simulink model "sm_DDPG_Training_Circuit_h4"  (R2022b)
settings: Solver=VariableStepAuto  StartTime=0.0  StopTime=2000  RelTol=1e-3
values from neighbouring files (symbols this model uses):
  areaFinEvap = 0.05    [pramInit.m]
  areaRoofRoom1 = roofArea/4    [pramInit.m]
  areaRoofRoom2 = roofArea/4    [pramInit.m]
  areaRoofRoom3 = roofArea/4    [pramInit.m]
  areaRoofRoom4 = roofArea/4    [pramInit.m]
  areaWallRoom1 = (lenHouse*3/5 *htHouse+widHouse*2/3*htHouse) - areaWindowRoom1    (= 95.6666666667)    [pramInit.m]
  areaWallRoom2 = (lenHouse*3/5*htHouse+widHouse/3*htHouse) - areaWindowRoom2    (= 83.3333333333)    [pramInit.m]
  areaWallRoom3 = (lenHouse*2/5*htHouse+widHouse*2/3*htHouse) - areaWindowRoom3    (= 72.6666666667)    [pramInit.m]
  areaWallRoom4 = (lenHouse*2/5*htHouse+widHouse/3*htHouse) - areaWindowRoom4    (= 59.3333333333)    [pramInit.m]
  areaWindowRoom1 = 3 * 1 *1    (= 3)    [pramInit.m]
  areaWindowRoom2 = 2 * 1 *1    (= 2)    [pramInit.m]
  areaWindowRoom3 = 2* 1 *1    (= 2)    [pramInit.m]
  areaWindowRoom4 = 2 * 1 *1    (= 2)    [pramInit.m]
  diaCond = 0.014    [pramInit.m]
  diaEvap = 0.126    [pramInit.m]
  diaGroundLoop = 0.032    [pramInit.m]
  diaOuterCond = 0.0158    [pramInit.m]
  diaOuterEvap = 0.1344    [pramInit.m]
  diaRadiatorPipe = 0.0125    [pramInit.m]
  htCondDuct = 0.3    [pramInit.m]
  htEvapDuct = 2.5    [pramInit.m]
  kTube = 400    [pramInit.m]
  leakRoofPercent = 0.1    [pramInit.m]
  leakWallPercent = 0.15    [pramInit.m]
  leakWinPercent = 0.2    [pramInit.m]
  numFinsEvap = 90    [pramInit.m]
  numTubeRowsCond = 20    [pramInit.m]
  numTubeRowsEvap = 400    [pramInit.m]
  numTubesPerRowCond = 10    [pramInit.m]
  numTubesPerRowEvap = 20    [pramInit.m]
  qGroundLoopPump = 18    [pramInit.m]
  roofDensity = 32    [pramInit.m]
  thkRoof = 0.2    [pramInit.m]
  thkWall = 0.2    [pramInit.m]
  thkWindow = 0.01    [pramInit.m]
  tInitHW = 50    [pramInit.m]
  tRoom = 23    [pramInit.m]
  Ts = hyper_agent_sample_time    [code_DDPG_Training.m]    (also in code_Experimental_Setup.m = 1)
  wallDensity = 1920    [pramInit.m]
  wCondDuct = 1.6    [pramInit.m]
  wEvapDuct = 0.96    [pramInit.m]
  windowDensity = 2700    [pramInit.m]
undefined symbols (not defined in the file or in its folder): DiscIntNeverNeededParam
libraries: fl_lib x144, nesl_utility x27, SimscapeFluids_lib x15, simulink x3, rllib x1
(part 1 of 4)
settings Model: Creator=rajeshs  LastModifiedBy=xmyci
settings SolverCC: AlgebraicLoopSolver=LineSearch
settings DebuggingCC: UnconnectedInputMsg=warning  UnconnectedOutputMsg=warning  UnconnectedLineMsg=warning  SFMachineParentedDataDiag=warning
settings ModelReferenceCC: EnableRefExpFcnMdlSchedulingChecks=on
settings SFSimCC: CustomCodeUndefinedFunction=UseInterfaceOnly
settings RTWCC: DLArmComputeVersion=19.05

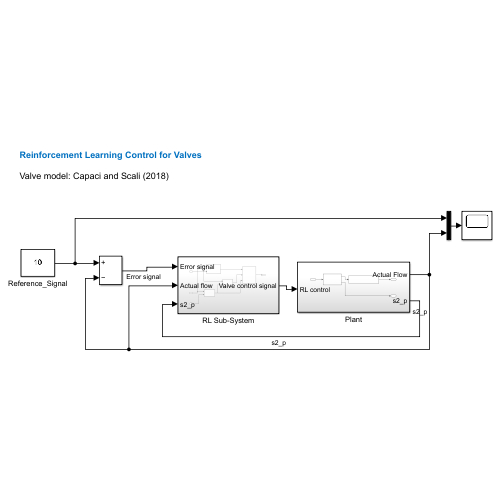
[thumbnail: Simulink's stored preview of the top-level diagram]
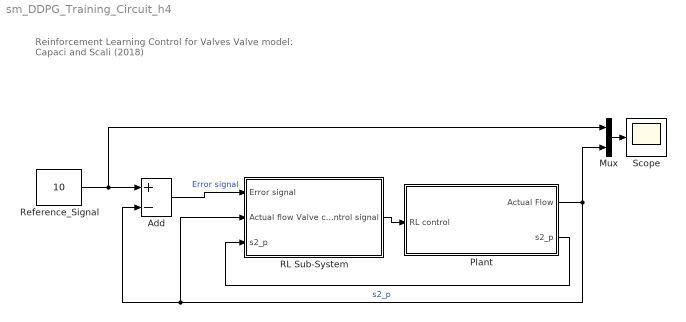
== system sm_DDPG_Training_Circuit_h4 ==
  note: Reinforcement Learning Control for Valves
      |
      | Valve model: Capaci and Scali (2018)
  Add : Sum  Inputs=+-
  Mux : Mux  Inputs=2
  Plant : Subsystem
  RL Sub-System : Subsystem
  Reference_Signal : Constant  Value=10
  Scope : Scope
  wires:
  Mux/1 -> Scope/1
  Add/1 -> RL Sub-System/1(Error signal)  "Error signal"
  Plant/1(Actual Flow) -> Add/2, RL Sub-System/2(Actual flow), Mux/2  "s2_p"
  Reference_Signal/1 -> Mux/1, Add/1
  RL Sub-System/1(Valve control signal) -> Plant/1(RL control)
  Plant/2(s2_p) -> RL Sub-System/3(s2_p)

== system sm_DDPG_Training_Circuit_h4/Plant ==
  RL control : Inport
  Non-linear Valve model : Subsystem
  Process : Subsystem
  Actual Flow : Outport  VectorParamsAs1DForOutWhenUnconnected=off
  s2_p : Outport  Port=2  VectorParamsAs1DForOutWhenUnconnected=off
  wires:
  Non-linear Valve model/1(ValveOutput) -> Process/1(Valve control)
  Process/1(Controlled_Flow) -> Actual Flow/1  "Actual Flow"
  RL control/1 -> Non-linear Valve model/1(ValveInput)
  Non-linear Valve model/2(S2_p) -> s2_p/1  "s2_p"

== system sm_DDPG_Training_Circuit_h4/RL Sub-System ==
  Error signal : Inport
  Actual flow : Inport  Port=2
  s2_p : Inport  Port=3
  Compute Rewards : Subsystem
  Observation vector : Subsystem
  RL Agent : rllib/RL Agent  Agent=agent  ExternalActionAsInput=off  ProvideLastAction=off  ProvideCumRwd=off  TreatAsDirectFeedthrough=on  UseStrictObservationDataTypes=off
  Stop-simulation : Subsystem
  Valve control signal : Outport  VectorParamsAs1DForOutWhenUnconnected=off
  wires:
  Stop-simulation/1(STOP) -> RL Agent/3, Compute Rewards/2(exceeds flow)
  Error signal/1 -> Compute Rewards/1(error), Observation vector/2(Error signal)
  Compute Rewards/1(reward) -> RL Agent/2
  Observation vector/1(Observation vector) -> RL Agent/1
  RL Agent/1 -> Valve control signal/1
  Actual flow/1 -> Observation vector/1(Actual flow), Stop-simulation/1(Actual flow)
  s2_p/1 -> Stop-simulation/2(s2_p)

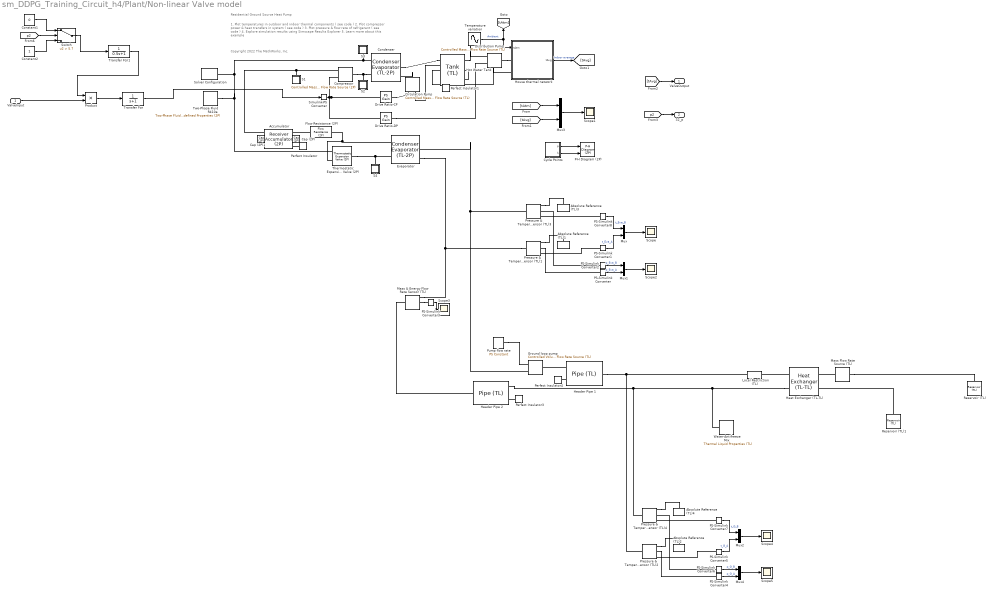
== system sm_DDPG_Training_Circuit_h4/Plant/Non-linear Valve model ==
  note: Copyright 2022 The MathWorks, Inc.
  note: Residential Ground Source Heat Pump
  note: 1. Plot temperatures in outdoor and indoor thermal components ( see code )
      | 2. Plot compressor power & heat transfers in system ( see code )
      | 3. Plot pressure & flow rate of refrigerant ( see code )
      | 4. Explore simulation results using Simscape Results Explorer
      | 5. Learn more about this example
  ValveInput : Inport
  Absolute Reference (TL){1..4} (4 alike) : fl_lib/Thermal Liquid/Elements/Absolute Reference (TL)
  Accumulator : SimscapeFluids_lib/Two-Phase Fluid/Tanks & Accumulators/Receiver Accumulator (2P)  volume=0.02 m^3  tank_area=0.5 m^2  area_AV=pi * diaEvap^2 / 4 m^2  area_BV=pi * diaEvap^2 / 4 m^2  area_AL=pi * diaEvap^2 / 4 m^2  area_BL=pi * diaEvap^2 / 4 m^2  V_frac_error=simscape.enum.assert.action.none  V_frac_min=0.05  V_frac_max=0.95  V_frac_smooth=0.001  p_crit_error=simscape.enum.assert.action.error  hc_vap=10 W/(m^2*K)  hc_liq=20 W/(m^2*K)  receiver_accumulator_energy_spec=fluids.two_phase_fluid.enum.receiver_accumulator_energy_spec.enthalpy  p_init=0.3 MPa  T_init=293.15 K  M_frac_init=0.5  V_frac_init=0.1 %L_init  h_init=436 kJ/kg  u_init=1500 kJ/kg  tau_vap_cond=1 s
      settings: InternalSimscapePortConfiguration="{\"Bottom\":[],\"Left\":[{\"id\":\"AV\",\"label\":\"AV\",\"type\":\"foundation.two_phase_fluid.two_phase_fluid\"},{\"id\":\"AL\",\"label\":\"AL\",\"type\":\"foundation.two_phase_fluid.two_phase_fluid\"},{\"id\":\"H\",\"label\":\"H\",\"type\":\"foundation.thermal.thermal\"}],\"Right\":[{\"id\":\"BV\",\"label\":\"BV\",\"type\":\"foundation.two_phase_fluid.two_phase_fluid\"},{\"id\":\"BL\",\"label\":\"BL\",\"type\":\"foundation.two_phase_fluid.two_phase_fluid\"},{\"id\":\"L\",\"label\":\"L\",\"type\":\"output\"}],\"Top\":[]}"
  Cap (2P) : fl_lib/Two-Phase Fluid/Elements/Cap (2P)  p_specify=off  p_priority=None  p=0.101325 MPa  p_nominal_specify=off  p_nominal_unit=MPa  p_nominal_value=1  u_specify=off  u_priority=None  u=1500 kJ/kg  u_nominal_specify=off  u_nominal_unit=kJ/kg  u_nominal_value=1
      settings: InternalSimscapePortConfiguration="{\"Bottom\":[],\"Left\":[{\"id\":\"A\",\"label\":\"\",\"type\":\"foundation.two_phase_fluid.two_phase_fluid\"}],\"Right\":[],\"Top\":[]}"
  Cap (2P)1 : fl_lib/Two-Phase Fluid/Elements/Cap (2P)  p_specify=off  p_priority=None  p=0.101325 MPa  p_nominal_specify=off  p_nominal_unit=MPa  p_nominal_value=1  u_specify=off  u_priority=None  u=1500 kJ/kg  u_nominal_specify=off  u_nominal_unit=kJ/kg  u_nominal_value=1
      settings: InternalSimscapePortConfiguration="{\"Bottom\":[],\"Left\":[{\"id\":\"A\",\"label\":\"\",\"type\":\"foundation.two_phase_fluid.two_phase_fluid\"}],\"Right\":[],\"Top\":[]}"
  Circulation Pump : fl_lib/Thermal Liquid/Sources/Controlled Mass Flow Rate Source (TL)  area=0.01 m^2
      settings: InternalSimscapePortConfiguration="{\"Bottom\":[],\"Left\":[{\"id\":\"A\",\"label\":\"A\",\"type\":\"foundation.thermal_liquid.thermal_liquid\"},{\"id\":\"M\",\"label\":\"M\",\"type\":\"input\"}],\"Right\":[{\"id\":\"B\",\"label\":\"B\",\"type\":\"foundation.thermal_liquid.thermal_liquid\"}],\"Top\":[]}"
  Compressor : fl_lib/Two-Phase Fluid/Sources/Controlled Mass Flow Rate Source (2P)  power_spec=foundation.enum.power_spec.isentropic  area_A=pi * diaCond^2 /4 m^2  area_B=pi * diaCond^2 /4 m^2
      settings: InternalSimscapePortConfiguration="{\"Bottom\":[],\"Left\":[{\"id\":\"A\",\"label\":\"A\",\"type\":\"foundation.two_phase_fluid.two_phase_fluid\"},{\"id\":\"M\",\"label\":\"M\",\"type\":\"input\"}],\"Right\":[{\"id\":\"B\",\"label\":\"B\",\"type\":\"foundation.two_phase_fluid.two_phase_fluid\"}],\"Top\":[]}"
  Condenser : SimscapeFluids_lib/Fluid Network Interfaces/Heat Exchangers/Condenser Evaporator (TL-2P)  flow_arrangement=fluids.interfaces.heat_exchangers.enum.FlowArrangementTL2P.Counter  cross_flow_arrangement=fluids.interfaces.heat_exchangers.enum.CrossFlowArrangementTL2P.UnmixedUnmixed  R_wall=log(diaOuterCond/diaCond) / (2*pi*kTube*wCondDuct*numTubeRowsCond*numTubesPerRowCond) K/kW  area_A1=wCondDuct * htCondDuct m^2  area_B1=wCondDuct * htCondDuct m^2  area_A2=pi * diaCond^2 /4 m^2  area_B2=pi * diaCond^2 /4 m^2  flow_geometry_TL=fluids.interfaces.heat_exchangers.enum.FlowGeometryTL.AcrossTubeBank  tube_num_TL=25  tube_length_TL=1 m  tube_cross_section_TL=fluids.interfaces.heat_exchangers.enum.TubeCrossSection.Circular  tube_diameter_TL=0.05 m  tube_width_TL=0.05 m  tube_height_TL=0.05 m  tube_inner_diameter_TL=0.05 m  tube_outer_diameter_TL=0.1 m  tube_flow_area_TL=0.002 m^2  tube_wetted_perimeter_TL=0.15 m  tube_heat_perimeter_TL=0.15 m  tube_pressure_loss_spec_TL=fluids.interfaces.heat_exchangers.enum.TubePressureLossSpec.Haaland  tube_loss_coeff_TL=10  tube_length_add_TL=0.1 m  tube_roughness_pressure_TL=15e-6 m  tube_Re_lam_pressure_TL=2000  tube_Re_tur_pressure_TL=4000  tube_shape_factor_generic_TL=64  tube_heat_coeff_spec_TL=fluids.interfaces.heat_exchangers.enum.TubeHeatCoeffSpec.Gneilinski  tube_colburn_coeff_TL=[.023, .8, .33]  tube_roughness_heat_TL=15e-6 m  tube_Re_lam_heat_TL=2000  tube_Re_tur_heat_TL=4000  tube_Nu_lam_generic_TL=3.66  bank_arrangement_TL=fluids.interfaces.heat_exchangers.enum.BankArrangement.Inline  bank_num_rows_TL=numTubeRowsCond  bank_tubes_per_row_TL=numTubesPerRowCond  bank_width_TL=wCondDuct m  bank_tube_diameter_TL=diaCond m  bank_longitudinal_pitch_TL=longPitchCond m  bank_transverse_pitch_TL=transPitchCond m  bank_pressure_loss_spec_TL=fluids.interfaces.heat_exchangers.enum.BankPressureLossSpec.Martin  bank_euler_TL=10  bank_heat_coeff_spec_TL=fluids.interfaces.heat_exchangers.enum.BankHeatCoeffSpec.Martin  bank_colburn_coeff_TL=[.27, .63, .36]  generic_flow_area_TL=0.01 m^2  generic_heat_area_TL=2 m^2  generic_volume_TL=0.05 m^3  generic_loss_coeff_TL=10  generic_colburn_coeff_TL=[.023, .8, .33]  fouling_factor_TL=0.1 K*m^2/kW  fin_area_TL=0.02 m^2  fin_efficiency_TL=0.5  p_init_TL=pInitHW MPa  T_init_TL=tInitHW degC  tube_num_2P=1  tube_length_2P=wCondDuct * numTubeRowsCond * numTubesPerRowCond m  tube_cross_section_2P=fluids.interfaces.heat_exchangers.enum.TubeCrossSection.Circular  tube_diameter_2P=diaCond m  tube_width_2P=0.05 m  tube_height_2P=0.05 m  tube_inner_diameter_2P=0.05 m  tube_outer_diameter_2P=0.1 m  tube_flow_area_2P=0.002 m^2  tube_wetted_perimeter_2P=0.15 m  tube_heat_perimeter_2P=0.15 m  tube_pressure_loss_spec_2P=fluids.interfaces.heat_exchangers.enum.TubePressureLossSpec2P.Haaland  tube_loss_coeff_2P=10  tube_length_add_2P=0.1 * numTubeRowsCond * numTubesPerRowCond m  tube_roughness_pressure_2P=15e-6 m  tube_Re_lam_pressure_2P=2000  tube_Re_tur_pressure_2P=4000  tube_shape_factor_generic_2P=64  tube_heat_coeff_spec_2P=fluids.interfaces.heat_exchangers.enum.TubeHeatCoeffSpec2P.GneilinskiCavalliniZecchin  tube_colburn_coeff_liq_2P=[.023, .8, .33]  tube_colburn_coeff_mix_2P=[.05, .8, .33]  tube_colburn_coeff_vap_2P=[.023, .8, .33]  tube_roughness_heat_2P=15e-6 m  tube_Re_lam_heat_2P=2000  tube_Re_tur_heat_2P=4000  tube_Nu_lam_generic_2P=3.66  fouling_factor_2P=0.1 K*m^2/kW  fin_area_2P=0 m^2  fin_efficiency_2P=0.5  energy_spec_2P=foundation.enum.energy_spec.enthalpy  p_init_2P=pInitCond MPa  T_init_2P=293.15 K  x_init_2P=x_init  alpha_init_2P=0.5  h_init_2P=enthalpyInitCond kJ/kg  u_init_2P=1500 kJ/kg
      settings: InternalSimscapePortConfiguration="{\"Bottom\":[],\"Left\":[{\"id\":\"A1\",\"label\":\"A1\",\"type\":\"foundation.thermal_liquid.thermal_liquid\"},{\"id\":\"B1\",\"label\":\"B1\",\"type\":\"foundation.thermal_liquid.thermal_liquid\"}],\"Right\":[{\"id\":\"A2\",\"label\":\"A2\",\"type\":\"foundation.two_phase_fluid.two_phase_fluid\"},{\"id\":\"B2\",\"label\":\"B2\",\"type\":\"foundation.two_phase_fluid.two_phase_fluid\"}],\"Top\":[{\"id\":\"Z\",\"label\":\"Z\",\"type\":\"output\"}]}"
  Constant1 : Constant  Value=0
  Constant2 : Constant
  Cycle Points : Subsystem
  Distribution Pump : fl_lib/Thermal Liquid/Sources/Controlled Mass Flow Rate Source (TL)  area=0.01 m^2
      settings: InternalSimscapePortConfiguration="{\"Bottom\":[],\"Left\":[{\"id\":\"A\",\"label\":\"A\",\"type\":\"foundation.thermal_liquid.thermal_liquid\"},{\"id\":\"M\",\"label\":\"M\",\"type\":\"input\"}],\"Right\":[{\"id\":\"B\",\"label\":\"B\",\"type\":\"foundation.thermal_liquid.thermal_liquid\"}],\"Top\":[]}"
  Drive Ratio-CP : fl_lib/Physical Signals/Functions/PS Gain  gain=30
  Drive Ratio-DP : fl_lib/Physical Signals/Functions/PS Gain  gain=90
  Evaporator : SimscapeFluids_lib/Fluid Network Interfaces/Heat Exchangers/Condenser Evaporator (TL-2P)  flow_arrangement=fluids.interfaces.heat_exchangers.enum.FlowArrangementTL2P.Cross  cross_flow_arrangement=fluids.interfaces.heat_exchangers.enum.CrossFlowArrangementTL2P.UnmixedUnmixed  R_wall=log(diaOuterEvap/diaEvap) / (2*pi*kTube*htEvapDuct*numTubeRowsEvap*numTubesPerRowEvap) K/kW  area_A1=wEvapDuct * htEvapDuct m^2  area_B1=wEvapDuct * htEvapDuct m^2  area_A2=pi * diaEvap^2 / 4 m^2  area_B2=pi * diaEvap^2 / 4 m^2  flow_geometry_TL=fluids.interfaces.heat_exchangers.enum.FlowGeometryTL.AcrossTubeBank  tube_num_TL=25  tube_length_TL=1 m  tube_cross_section_TL=fluids.interfaces.heat_exchangers.enum.TubeCrossSection.Circular  tube_diameter_TL=0.05 m  tube_width_TL=0.05 m  tube_height_TL=0.05 m  tube_inner_diameter_TL=0.05 m  tube_outer_diameter_TL=0.1 m  tube_flow_area_TL=0.002 m^2  tube_wetted_perimeter_TL=0.15 m  tube_heat_perimeter_TL=0.15 m  tube_pressure_loss_spec_TL=fluids.interfaces.heat_exchangers.enum.TubePressureLossSpec.Haaland  tube_loss_coeff_TL=10  tube_length_add_TL=0.1 m  tube_roughness_pressure_TL=15e-6 m  tube_Re_lam_pressure_TL=2000  tube_Re_tur_pressure_TL=4000  tube_shape_factor_generic_TL=64  tube_heat_coeff_spec_TL=fluids.interfaces.heat_exchangers.enum.TubeHeatCoeffSpec.Gneilinski  tube_colburn_coeff_TL=[.023, .8, .33]  tube_roughness_heat_TL=15e-6 m  tube_Re_lam_heat_TL=2000  tube_Re_tur_heat_TL=4000  tube_Nu_lam_generic_TL=3.66  bank_arrangement_TL=fluids.interfaces.heat_exchangers.enum.BankArrangement.Staggered  bank_num_rows_TL=numTubeRowsEvap  bank_tubes_per_row_TL=numTubesPerRowEvap  bank_width_TL=htEvapDuct m  bank_tube_diameter_TL=diaEvap m  bank_longitudinal_pitch_TL=longPitchEvap m  bank_transverse_pitch_TL=transPitchEvap m  bank_pressure_loss_spec_TL=fluids.interfaces.heat_exchangers.enum.BankPressureLossSpec.Martin  bank_euler_TL=10  bank_heat_coeff_spec_TL=fluids.interfaces.heat_exchangers.enum.BankHeatCoeffSpec.Martin  bank_colburn_coeff_TL=[.27, .63, .36]  generic_flow_area_TL=0.01 m^2  generic_heat_area_TL=2 m^2  generic_volume_TL=0.05 m^3  generic_loss_coeff_TL=10  generic_colburn_coeff_TL=[.023, .8, .33]  fouling_factor_TL=0.1 K*m^2/kW  fin_area_TL=numFinsEvap*areaFinEvap m^2  fin_efficiency_TL=0.5  p_init_TL=0.101325 MPa  T_init_TL=tInitGround degC  tube_num_2P=1  tube_length_2P=htEvapDuct * numTubeRowsEvap * numTubesPerRowEvap m  tube_cross_section_2P=fluids.interfaces.heat_exchangers.enum.TubeCrossSection.Circular  tube_diameter_2P=diaEvap m  tube_width_2P=0.05 m  tube_height_2P=0.05 m  tube_inner_diameter_2P=0.05 m  tube_outer_diameter_2P=0.1 m  tube_flow_area_2P=0.002 m^2  tube_wetted_perimeter_2P=0.15 m  tube_heat_perimeter_2P=0.15 m  tube_pressure_loss_spec_2P=fluids.interfaces.heat_exchangers.enum.TubePressureLossSpec2P.Haaland  tube_loss_coeff_2P=10  tube_length_add_2P=0.5 * htEvapDuct * numTubeRowsEvap * numTubesPerRowEvap m  tube_roughness_pressure_2P=15e-6 m  tube_Re_lam_pressure_2P=2000  tube_Re_tur_pressure_2P=4000  tube_shape_factor_generic_2P=64  tube_heat_coeff_spec_2P=fluids.interfaces.heat_exchangers.enum.TubeHeatCoeffSpec2P.GneilinskiCavalliniZecchin  tube_colburn_coeff_liq_2P=[.023, .8, .33]  tube_colburn_coeff_mix_2P=[.05, .8, .33]  tube_colburn_coeff_vap_2P=[.023, .8, .33]  tube_roughness_heat_2P=15e-6 m  tube_Re_lam_heat_2P=2000  tube_Re_tur_heat_2P=4000  tube_Nu_lam_generic_2P=3.66  fouling_factor_2P=0.1 K*m^2/kW  fin_area_2P=0 m^2  fin_efficiency_2P=0.5  energy_spec_2P=foundation.enum.energy_spec.enthalpy  p_init_2P=pInitEvap MPa  T_init_2P=293.15 K  x_init_2P=0.5  alpha_init_2P=0.5  h_init_2P=enthalpyInitEvap kJ/kg  u_init_2P=1500 kJ/kg
      settings: InternalSimscapePortConfiguration="{\"Bottom\":[],\"Left\":[{\"id\":\"A1\",\"label\":\"A1\",\"type\":\"foundation.thermal_liquid.thermal_liquid\"},{\"id\":\"B1\",\"label\":\"B1\",\"type\":\"foundation.thermal_liquid.thermal_liquid\"}],\"Right\":[{\"id\":\"A2\",\"label\":\"A2\",\"type\":\"foundation.two_phase_fluid.two_phase_fluid\"},{\"id\":\"B2\",\"label\":\"B2\",\"type\":\"foundation.two_phase_fluid.two_phase_fluid\"}],\"Top\":[{\"id\":\"Z\",\"label\":\"Z\",\"type\":\"output\"}]}"
  Flow Resistance (2P) : fl_lib/Two-Phase Fluid/Elements/Flow Resistance (2P)  delta_p_nominal=0.001 MPa  mdot_nominal=0.225 kg/s  v_nominal=0 m^3/kg  area=pi * diaEvap^2 / 4 m^2  laminar_fraction=1e-3
      settings: InternalSimscapePortConfiguration="{\"Bottom\":[],\"Left\":[{\"id\":\"A\",\"label\":\"A\",\"type\":\"foundation.two_phase_fluid.two_phase_fluid\"}],\"Right\":[{\"id\":\"B\",\"label\":\"B\",\"type\":\"foundation.two_phase_fluid.two_phase_fluid\"}],\"Top\":[]}"
  Ground loop pump : fl_lib/Thermal Liquid/Sources/Controlled Volumetric Flow Rate Source (TL)  area=wEvapDuct * htEvapDuct m^2
      settings: InternalSimscapePortConfiguration="{\"Bottom\":[],\"Left\":[{\"id\":\"A\",\"label\":\"A\",\"type\":\"foundation.thermal_liquid.thermal_liquid\"},{\"id\":\"V\",\"label\":\"V\",\"type\":\"input\"}],\"Right\":[{\"id\":\"B\",\"label\":\"B\",\"type\":\"foundation.thermal_liquid.thermal_liquid\"}],\"Top\":[]}"
  Header Pipe 1 : SimscapeFluids_lib/Thermal Liquid/Pipes & Fittings/Pipe (TL)  dynamic_compressibility=simscape.enum.onoff.on  inertia=simscape.enum.onoff.off  num_segments=1  pipe_length=lenHeaderPipe1 m  area=pi * diaGroundLoop^2 / 4 m^2  wall_spec=fluids.thermal_liquid.pipes_fittings.enum.wall_spec.rigid  Dh=diaGroundLoop m  wall_compliance=1.2e-6 m/MPa  wall_time_constant=0.01 s  elevation_spec=foundation.enum.constant_variable.constant  elevation_gain=0 m  g=9.81 m/s^2  pressure_loss_spec=fluids.thermal_liquid.pipes_fittings.enum.PressureLossSpec.Haaland  local_pressure_loss_spec=fluids.thermal_liquid.pipes_fittings.enum.LocalLossSpec.AggregateLength  length_add=1 m  loss_coefficient=0.1  roughness=15e-6 m  Re_friction_TLU=[400, 1000, 1500, 3000, 4000, 6000, 10000, 20000, 40000, 60000, 100000, 100000000]  friction_factor_TLU=[.264, .112, .071, .0417, .0387, .0268, .025, .0232, .0226, .022, .0214, .0214]  shape_factor=64  Re_lam=2000  Re_tur=4000  mdot_nominal=[.1, 1] kg/s  p_diff_nominal=[.001, .01] MPa  mdot_threshold=1e-6 kg/s  heat_transfer_spec=fluids.thermal_liquid.pipes_fittings.enum.HeatTransferSpec.Gnielinski  mdot_nominal_heat=[.1, 1] kg/s  T_in_nominal=[293.15, 293.15] K  T_out_nominal=[300, 300] K  p_in_nominal_heat=[.101325, .101325] MPa  T_wall_nominal=[303.15, 303.15] K  a_coeff=0.023  b_Re_power=0.8  c_Pr_power=0.4  Nu_lam=3.66  Re_Colburn_TLU=[100, 150, 1000]  Colburn_factor_TLU=[.019, .013, .002]  Re_Nu_TLU=[100, 150, 1000]  Pr_Nu_TLU=[1, 10]  Nu_TLU=[3.72, 4.21; 3.75, 4.44; 4.21, 7.15]  T0_vec=tInitGround degC  p0_vec=0.101325 MPa  mdot0=0.1 kg/s
  Header Pipe 2 : SimscapeFluids_lib/Thermal Liquid/Pipes & Fittings/Pipe (TL)  dynamic_compressibility=simscape.enum.onoff.on  inertia=simscape.enum.onoff.off  num_segments=1  pipe_length=lenHeaderPipe2 m  area=pi * diaGroundLoop^2 / 4 m^2  wall_spec=fluids.thermal_liquid.pipes_fittings.enum.wall_spec.rigid  Dh=diaGroundLoop m  wall_compliance=1.2e-6 m/MPa  wall_time_constant=0.01 s  elevation_spec=foundation.enum.constant_variable.constant  elevation_gain=0 m  g=9.81 m/s^2  pressure_loss_spec=fluids.thermal_liquid.pipes_fittings.enum.PressureLossSpec.Haaland  local_pressure_loss_spec=fluids.thermal_liquid.pipes_fittings.enum.LocalLossSpec.AggregateLength  length_add=1 m  loss_coefficient=0.1  roughness=15e-6 m  Re_friction_TLU=[400, 1000, 1500, 3000, 4000, 6000, 10000, 20000, 40000, 60000, 100000, 100000000]  friction_factor_TLU=[.264, .112, .071, .0417, .0387, .0268, .025, .0232, .0226, .022, .0214, .0214]  shape_factor=64  Re_lam=2000  Re_tur=4000  mdot_nominal=[.1, 1] kg/s  p_diff_nominal=[.001, .01] MPa  mdot_threshold=1e-6 kg/s  heat_transfer_spec=fluids.thermal_liquid.pipes_fittings.enum.HeatTransferSpec.Gnielinski  mdot_nominal_heat=[.1, 1] kg/s  T_in_nominal=[293.15, 293.15] K  T_out_nominal=[300, 300] K  p_in_nominal_heat=[.101325, .101325] MPa  T_wall_nominal=[303.15, 303.15] K  a_coeff=0.023  b_Re_power=0.8  c_Pr_power=0.4  Nu_lam=3.66  Re_Colburn_TLU=[100, 150, 1000]  Colburn_factor_TLU=[.019, .013, .002]  Re_Nu_TLU=[100, 150, 1000]  Pr_Nu_TLU=[1, 10]  Nu_TLU=[3.72, 4.21; 3.75, 4.44; 4.21, 7.15]  T0_vec=tInitGround degC  p0_vec=0.101325 MPa  mdot0=0.1 kg/s
  Heat Exchanger (TL-TL) : SimscapeFluids_lib/Fluid Network Interfaces/Heat Exchangers/Heat Exchanger (TL-TL)  hex_type=fluids.interfaces.enum.flow_arrangement_spec.parallel_counter  shell_num=1  cross_type=fluids.interfaces.enum.cross_flow_heat_exchanger_TL_TL_spec.mixed_mixed  NTU_TLU=[.5, 1, 2, 3, 4, 5]  CR_TLU=[0, .25, .5, .75, 1]  eff_TLU=[.3, .3, .3, .3, .3; .6, .55, .5, .47, .43; .85, .76, .68, .61, .55; .94, .83, .72, .65, .58; .98, .86, .75, .66, .58; .99, .86, .75, .66, .58]  wall_thermal_dynamics=simscape.enum.onoff.off  thermal_mass_wall=447 J/K  R_wall=1.6e-4 K/W  min_flow_area_1=0.01 m^2  Dh_press_1=0.1 m  liquid_volume_1=0.01 m^3  Re_lam_1=2000  Re_tur_1=4000  pressure_loss_spec_1=fluids.interfaces.enum.pressure_loss_spec.constant  pressure_loss_coeff_1=0.1  length_press_1=1 m  length_add_1=0.1 m  roughness_1=15e-6 m  Re_friction_TLU_1=[400, 1000, 1500, 3000, 4000, 6000, 10000, 20000, 40000, 60000, 100000, 100000000]  friction_factor_TLU_1=[.264, .112, .071, .0417, .0387, .0268, .025, .0232, .0226, .022, .0214, .0214]  shape_factor_1=64  Re_Euler_TLU_1=[50, 500, 1000, 2000]  Euler_TLU_1=[4.4505, .6864, .4791, .3755]  heat_transfer_spec_1=fluids.interfaces.enum.heat_transfer_spec.constant  heat_transfer_area_1=0.4 m^2  heat_coeff_1=100 W/(K*m^2)  length_heat_1=1 m  Nu_lam_1=3.66  Re_Colburn_TLU_1=[100, 150, 1000]  Colburn_factor_TLU_1=[.019, .013, .002]  Re_Nu_TLU_1=[100, 150, 1000]  Pr_Nu_TLU_1=[1, 10]  Nu_TLU_1=[3.72, 4.21; 3.75, 4.44; 4.21, 7.15]  fouling_factor_1=1e-4 K*m^2/W  min_heat_coeff_1=5 W/(K*m^2)  min_flow_area_2=0.01 m^2  Dh_press_2=0.1 m  liquid_volume_2=0.01 m^3  Re_lam_2=2000  Re_tur_2=4000  pressure_loss_spec_2=fluids.interfaces.enum.pressure_loss_spec.constant  pressure_loss_coeff_2=0.1  length_press_2=1 m  length_add_2=0.1 m  roughness_2=15e-6 m  Re_friction_TLU_2=[400, 1000, 1500, 3000, 4000, 6000, 10000, 20000, 40000, 60000, 100000, 100000000]  friction_factor_TLU_2=[.264, .112, .071, .0417, .0387, .0268, .025, .0232, .0226, .022, .0214, .0214]  shape_factor_2=64  Re_Euler_TLU_2=[50, 500, 1000, 2000]  Euler_TLU_2=[4.4505, .6864, .4791, .3755]  heat_transfer_spec_2=fluids.interfaces.enum.heat_transfer_spec.constant  heat_transfer_area_2=0.4 m^2  heat_coeff_2=100 W/(K*m^2)  length_heat_2=1 m  Nu_lam_2=3.66  Re_Colburn_TLU_2=[100, 150, 1000]  Colburn_factor_TLU_2=[.019, .013, .002]  Re_Nu_TLU_2=[100, 150, 1000]  Pr_Nu_TLU_2=[1, 10]  Nu_TLU_2=[3.72, 4.21; 3.75, 4.44; 4.21, 7.15]  fouling_factor_2=1e-4 K*m^2/W  min_heat_coeff_2=5 W/(K*m^2)  dynamic_compressibility_1=simscape.enum.onoff.on  T0_1=293.15 K  p0_1=0.101325 MPa  dynamic_compressibility_2=simscape.enum.onoff.on  T0_2=293.15 K  p0_2=0.101325 MPa  mdot1_TLU=[.3, .5, .6, .7, 1, 1.4, 1.9, 2.3] kg/s  mdot2_TLU=[.3, .5, 1, 1.3, 1.7, 2, 2.6, 3.3] kg/s  SD_TLU=[.324, .3533, .404, .4253, .4333, .4373, .4453, .4533; .3813, .424, .496, .5307, .544, .5547, .5693, .5787; .4267, .4827, .5813, .6173, .6413, .6573, .672, .6827; .4613, .528, .64, .6987, .7267, .7467, .7707, .7853; .5533, .6467, .8227, .928, .9853, 1.0187, 1.0653, 1.0973; .58, .688, .8853, 1.0147, 1.08, 1.124, 1.176, 1.2147; .624, .7467, .992, 1.148, 1.244, 1.304, 1.3773, 1.4267; .656, .7907, 1.0667, 1.26, 1.376, 1.452, 1.548, 1.612] kW/K  Q_check=fluids.interfaces.enum.SD_max_check.warning  mdot_dp_TLU_1=[.3, .5, 1, 1.5, 2, 2.5] kg/s  p_diff_TLU_1=[3, 5, 10, 25, 35, 50] * 1e-3 MPa  T_ref_in_1=293.15 K  p_ref_in_1=0.101325 MPa  mdot_threshold_1=1e-3 kg/s  area_1=0.01 m^2  mdot_dp_TLU_2=[.3, .5, 1, 1.5, 2, 2.5] kg/s  p_diff_TLU_2=[3, 5, 10, 25, 35, 50] * 1e-3 MPa  T_ref_in_2=293.15 K  p_ref_in_2=0.101325 MPa  mdot_threshold_2=1e-3 kg/s  area_2=0.01 m^2
      settings: InternalSimscapePortConfiguration="{\"Bottom\":[],\"Left\":[{\"id\":\"A1\",\"label\":\"A1\",\"type\":\"foundation.thermal_liquid.thermal_liquid\"},{\"id\":\"B1\",\"label\":\"B1\",\"type\":\"foundation.thermal_liquid.thermal_liquid\"}],\"Right\":[{\"id\":\"A2\",\"label\":\"A2\",\"type\":\"foundation.thermal_liquid.thermal_liquid\"},{\"id\":\"B2\",\"label\":\"B2\",\"type\":\"foundation.thermal_liquid.thermal_liquid\"}],\"Top\":[]}"
  Hot Water Tank : SimscapeFluids_lib/Thermal Liquid/Tanks & Accumulators/Tank (TL)  num_inlet=fluids.thermal_liquid.tanks_accumulators.enum.NumInlet.Four  pressure_spec=foundation.enum.pressure_spec.atmospheric  tank_pressure=0.101325 MPa  volume_spec=fluids.thermal_liquid.tanks_accumulators.enum.TankVolumeSpec.Constant  tank_area=0.2 m^2  level_TLU=[0, 3, 5] m  volume_TLU=[0, 4, 6] m^3  inlet_height_A=0.1 m  inlet_area_A=0.01 m^2  inlet_heights_AB=[.1, .1] m  inlet_areas_AB=[.01, .01] m^2  inlet_heights_ABC=[.1, .1, .1] m  inlet_areas_ABC=[.01, .01, .01] m^2  inlet_heights_ABCD=0.1 * ones(1, 4) m  inlet_areas_ABCD=wCondDuct * htCondDuct * ones(1, 4) m^2  inlet_heights_ABCDE=0.1 * ones(1, 5) m  inlet_areas_ABCDE=0.01 * ones(1, 5) m^2  inlet_heights_ABCDEF=0.1 * ones(1, 6) m  inlet_areas_ABCDEF=0.01 * ones(1, 6) m^2  level_check=simscape.enum.assert.action.error  capacity_check=simscape.enum.assert.action.error  max_capacity=0.2 m^3  g=9.81 m/s^2  level_specify=on  level_priority=High  level=0.9 m  level_nominal_specify=off  level_nominal_unit=m  level_nominal_value=1  volume_specify=off  volume_priority=Low  volume=0.5 m^3  volume_nominal_specify=off  volume_nominal_unit=m^3  volume_nominal_value=1  mass_specify=off  mass_priority=None  mass=5000 kg  mass_nominal_specify=off  mass_nominal_unit=kg  mass_nominal_value=1  T_I_specify=on  T_I_priority=High  T_I=tInitHW degC  T_I_nominal_specify=off  T_I_nominal_unit=K  T_I_nominal_value=1
      settings: InternalSimscapePortConfiguration="{\"Bottom\":[{\"id\":\"H\",\"label\":\"H\",\"type\":\"foundation.thermal.thermal\"},{\"id\":\"T_out\",\"label\":\"T\",\"type\":\"output\"}],\"Left\":[{\"id\":\"A\",\"label\":\"A\",\"type\":\"foundation.thermal_liquid.thermal_liquid\"},{\"id\":\"B\",\"label\":\"B\",\"type\":\"foundation.thermal_liquid.thermal_liquid\"},{\"id\":\"C\",\"label\":\"C\",\"type\":\"foundation.thermal_liquid.thermal_liquid\"}],\"Right\":[{\"id\":\"D\",\"label\":\"D\",\"type\":\"foundation.thermal_liquid.thermal_liquid\"}],\"Top\":[{\"id\":\"V_out\",\"label\":\"V\",\"type\":\"output\"},{\"id\":\"L_out\",\"label\":\"L\",\"type\":\"output\"}]}"
  House thermal network : Subsystem
      mask Display:
      | plot([99.4454661849886;170.309218810871;170.309218810871;99.4454661849886;99.4454661849886], [212.827470386401;212.827470386401;127.790967235342;127.790967235342;212.827470386401])
      | plot([99.4454661849886;170.309218810871], [184.481969336048;184.481969336048])
      | plot([133.460067445412;133.460067445412], [184.481969336048;127.790967235342])
      | plot([241.172971436754;312.036724062636;312.036724062636;241.172971436754;241.172971436754], [212.827470386401;212.827470386401;127.790967235342;127.790967235342;212.827470386401])
      | plot([241.172971436754;312.036724062636], [184.481969336048;184.481969336048])
      | plot([275.187572697178;275.187572697178], [184.481969336048;127.790967235342])
      | plot([113.618216710165;42.7544640842825;368.727726163343;428.253278369084], [453.764229314402;255.34572196193;255.34572196193;453.764229314402])
      | plot([428.253278369084;499.117030994967], [453.764229314402;382.900476688519])
      | plot([113.618216710165;428.253278369084], [453.764229314402;453.764229314402])
      | plot([498.86507098563;499.368991004303], [382.900476688519;382.900476688519])
      | plot([482.109730364755;496.282480889931], [382.900476688519;382.900476688519])
      | plot([482.109730364755;374.396826373413], [382.900476688519;275.187572697178])
      | plot([482.109730364755;425.418728264049], [382.900476688519;439.591478789225])
      | plot([56.927214609459;56.927214609459;354.554975638166], [255.34572196193;56.927214609459;56.927214609459])
      | plot([354.554975638166;354.554975638166], [56.927214609459;255.34572196193])
      | plot([354.554975638166;482.109730364755;482.109730364755], [56.927214609459;184.481969336048;382.900476688519])
      | plot([397.073227213696;397.073227213696;439.591478789225;439.591478789225;397.073227213696], [170.309218810871;255.34572196193;297.86397353746;209.992920281366;170.309218810871])
      | plot([397.073227213696;439.591478789225], [227.000220911577;269.518472487107])
      | plot([419.749628053978;419.749628053978], [246.842071646824;192.985619651154])
  Local Restriction (TL) : fl_lib/Thermal Liquid/Elements/Local Restriction (TL)  restriction_type=foundation.enum.restriction_type.fixed  restriction_area=pi*0.05^2*0.1 m^2  min_area=1e-10 m^2  max_area=0.005 m^2  area=pi*0.1^2 m^2  Cd=0.7  pressure_recovery=1  Re_c=12
  Mass & Energy Flow Rate Sensor (TL) : fl_lib/Thermal Liquid/Sensors/Mass & Energy Flow Rate Sensor (TL)
      settings: InternalSimscapePortConfiguration="{\"Bottom\":[],\"Left\":[{\"id\":\"A\",\"label\":\"A\",\"type\":\"foundation.thermal_liquid.thermal_liquid\"}],\"Right\":[{\"id\":\"B\",\"label\":\"B\",\"type\":\"foundation.thermal_liquid.thermal_liquid\"},{\"id\":\"M\",\"label\":\"M\",\"type\":\"output\"},{\"id\":\"PHI\",\"label\":\"Phi\",\"type\":\"output\"}],\"Top\":[]}"
  Mass Flow Rate Source (TL) : fl_lib/Thermal Liquid/Sources/Mass Flow Rate Source (TL)  commanded_mass_flow=10 kg/s  area=0.01 m^2
      settings: InternalSimscapePortConfiguration="{\"Bottom\":[],\"Left\":[{\"id\":\"A\",\"label\":\"A\",\"type\":\"foundation.thermal_liquid.thermal_liquid\"}],\"Right\":[{\"id\":\"B\",\"label\":\"B\",\"type\":\"foundation.thermal_liquid.thermal_liquid\"}],\"Top\":[]}"
  Mux{,1..4} (5 alike) : Mux  Inputs=2
  P-H Diagram (2P) : SimscapeFluids_lib/Two-Phase Fluid/Utilities/P-H Diagram (2P)
  PS-Simulink Converter{,1..8} (9 alike) : nesl_utility/PS-Simulink Converter  PhysicalDomain=network_engine_domain  SubClassName=ps_output  LeftPortType=input  RightPortType=output  PseudoPeriodic=off  Frequencies=[]  VectorFormat=inherit  Unit=inherit  AffineConversion=off
  Perfect Insulator : fl_lib/Thermal/Thermal Elements/Perfect Insulator  T_specify=off  T_priority=None  T=0 K  T_nominal_specify=off  T_nominal_unit=K  T_nominal_value=1
  Perfect Insulator1 : fl_lib/Thermal/Thermal Elements/Perfect Insulator  T_specify=on  T_priority=None  T=tInitHW degC  T_nominal_specify=off  T_nominal_unit=K  T_nominal_value=1
  Perfect Insulator3 : fl_lib/Thermal/Thermal Elements/Perfect Insulator  T_specify=off  T_priority=None  T=0 K  T_nominal_specify=off  T_nominal_unit=K  T_nominal_value=1
  Perfect Insulator4 : fl_lib/Thermal/Thermal Elements/Perfect Insulator  T_specify=off  T_priority=None  T=0 K  T_nominal_specify=off  T_nominal_unit=K  T_nominal_value=1
  Pressure & Temperature Sensor (TL){1..4} (4 alike) : fl_lib/Thermal Liquid/Sensors/Pressure & Temperature Sensor (TL)
      settings: InternalSimscapePortConfiguration="{\"Bottom\":[],\"Left\":[{\"id\":\"A\",\"label\":\"A\",\"type\":\"foundation.thermal_liquid.thermal_liquid\"}],\"Right\":[{\"id\":\"B\",\"label\":\"B\",\"type\":\"foundation.thermal_liquid.thermal_liquid\"},{\"id\":\"P\",\"label\":\"P\",\"type\":\"output\"},{\"id\":\"T\",\"label\":\"T\",\"type\":\"output\"}],\"Top\":[]}"
  Product : Product
  Pump flow rate : fl_lib/Physical Signals/Sources/PS Constant  constant=qGroundLoopPump*49 lpm
  Reservoir (TL) : fl_lib/Thermal Liquid/Elements/Reservoir (TL)  pressure_spec=foundation.enum.pressure_spec.atmospheric  reservoir_pressure=0.101325 MPa  reservoir_temperature=310 K  area=0.01 m^2
  Reservoir (TL)1 : fl_lib/Thermal Liquid/Elements/Reservoir (TL)  pressure_spec=foundation.enum.pressure_spec.atmospheric  reservoir_pressure=0.101325 MPa  reservoir_temperature=300 K  area=0.01 m^2
  S1 : Subsystem
      settings: PortSchema="{\"entries\":[{\"content\":{\"sides\":[{\"content\":{\"connectorIds\":[]},\"type\":\"ConnectorPlacement.EquallySpacedRectSide\",\"uuid\":\"bdad09c6-2447-4c67-b82d-8a3c5cdf111f\"},{\"content\":{\"connectorIds\":[],\"side\":\"RIGHT\"},\"type\":\"ConnectorPlacement.EquallySpacedRectSide\",\"uuid\":\"4cbc956b-d91c-43cf-ae4b-b888705718b5\"},{\"content\":{\"connectorIds\":[],\"side\":\"TOP\"},\"type\":\"ConnectorPlacement.EquallySpacedRectSide\",\"uuid\":\"435bc899-fd44-4876-8d85-25be6407312a\"},{\"content\":{\"connectorIds\":[\"RConn1\"],\"side\":\"BOTTOM\"},\"type\":\"ConnectorPlacement.EquallySpacedRectSide\",\"uuid\":\"cca63654-a070-48e1-8fa2-13ef18996911\"}]},\"type\":\"ConnectorPlacement.EquallySpacedConnector\",\"uuid\":\"ad1db507-3712-4638-8577-d902b1cbac2d\"}],\"packageUris\":[\"http://schema.mathworks.com/mf0/Connector/R2020b\"],\"version\":\"1.0\"}"
      mask Display: disp(get_param(gcb, 'Name'))
  S2 : Subsystem
      mask Display: disp(get_param(gcb, 'Name'))
  S3 : Subsystem
      mask Display: disp(get_param(gcb, 'Name'))
  S4 : Subsystem
      mask Display: disp(get_param(gcb, 'Name'))
  Scope{,1..5} (6 alike) : Scope
  Simulink-PS Converter : nesl_utility/Simulink-PS Converter  PhysicalDomain=network_engine_domain  SubClassName=ps_input  LeftPortType=input  RightPortType=output  PseudoPeriodic=off  Frequencies=[]  NoiseDistribution=none  NoiseParameters=[]  Unit=kg/s  AffineConversion=off  FilteringAndDerivatives=provide  SimscapeFilterOrder=1  InputFilterTimeConstant=0.001  UdotUserProvided=0
  Solver Configuration : nesl_utility/Solver Configuration  PhysicalDomain=network_engine_domain  SubClassName=solver  LeftPortType=input  RightPortType=generic  Tones=[]  Harmonics=[]  SimulateNoise=off  Profile=off  UseLocalSampling=off  EnableSwitchedLinearOptims=on  FrequencyDomain=off  UseCCode=off  RelTol=0.001  AbsTol=1e-06  MinStep=1e-09  ToWorkspace=off  RevertToSquareIcSolve=off  NumHomotopyIterations=100  PhasorMode=off  PhasorModeNumHarmonics=1  ConsistencySolver=NEWTON_FTOL  IndexReductionMethod=DerivativeReplacement  DoDC=off  ResidualTolerance=1e-09  ConsistencyTolSource=GLOBAL  ConsistencyAbsTol=0.001  ConsistencyRelTol=0.001  ConsistencyTolFactor=0.001  UseLocalSolver=off  LocalSolverChoice=NE_BACKWARD_EULER_ADVANCER  ResolveIndetEquations=on  FunctionEvalNumThread=1  LocalSolverSampleTime=0.001  DoFixedCost=off  MaxNonlinIter=4  MaxModeIter=3  ComputeImpulses=off  ImpulseIterations=2  LinearAlgebra=auto  LinearAlgebraNumThread=0  EquationFormulation=NE_TIME_EF  DelaysMemoryBudget=1024  AutomaticFiltering=on  FilteringTimeConstant=0.001  PartitionStorageMethod=AS_NEEDED  PartitionMemoryBudget=1024  PartitionMethod=ROBUST
  Switch : Switch  Criteria=u2 > Threshold  Threshold=5.7  SaturateOnIntegerOverflow=off  InputSameDT=off
  Temperature variation : Sin  Amplitude=2  Bias=12  Frequency=2*pi/(24*3600)  SampleTime=0
  Thermostatic Expansion Valve (2P) : SimscapeFluids_lib/Two-Phase Fluid/Valves & Orifices/Flow Control Valves/Thermostatic Expansion Valve (2P)  valve_parameterization=fluids.two_phase_fluid.valves_orifices.flow_control_valves.enum.ThermostaticExpansionValveParameterization.Nominal  capacity_spec=fluids.two_phase_fluid.valves_orifices.flow_control_valves.enum.ThermostaticExpansionValveCapacitySpec.MassFlowRate  Q_nominal=nomQEvap kW  Q_max=maxQEvap kW  mdot_nominal=0.18 kg/s  mdot_max=1.5*0.18 kg/s  pressure_spec=fluids.two_phase_fluid.valves_orifices.flow_control_valves.enum.ThermostaticExpansionValvePressureSpec.SaturationTemperature  p_cond_nominal=1.5 MPa  p_evap_nominal=0.5 MPa  T_cond_nominal=50 degC  T_evap_nominal=-20 degC  delta_T_sub=tSubcool deltadegC  delta_T_nominal=tSuperheatNom deltadegC  delta_T_static=tSuperheatStatic deltadegC  mop=fluids.two_phase_fluid.valves_orifices.flow_control_valves.enum.ThermostaticExpansionValveMOP.Off  p_mop=0.5 MPa  T_mop=288.15 K  mdot_leak_fraction=1e-6  smoothing_factor=0.01  T_evap_out_TLU1=0 : 10 : 40 degC  p_bulb_TLU1=0.3 : 0.1 : 0.7 MPa  lift_TLU2=0 : 0.15 : 0.6 mm  p_evap_TLU2=0.3 : -0.05 : 0.1 MPa  lift_TLU3=0 : 0.15 : 0.6 mm  mdot_TLU3=0 : 0.015 : 0.06 kg/s  p_cond_ref=2 MPa  p_evap_ref=0.2 MPa  T_evap_out_ref=0 degC  delta_T_sub_ref=5 deltaK  pressure_equalization=fluids.two_phase_fluid.valves_orifices.flow_control_valves.enum.ThermostaticExpansionValveEqualization.Internal  bulb_dynamics=simscape.enum.onoff.off  tau_bulb=20 s  area=pi * diaEvap^2 / 4 m^2  B_lam=0.999  tau_x=0.1 s
      settings: InternalSimscapePortConfiguration="{\"Bottom\":[],\"Left\":[{\"id\":\"A\",\"label\":\"A\",\"type\":\"foundation.two_phase_fluid.two_phase_fluid\"}],\"Right\":[{\"id\":\"B\",\"label\":\"B\",\"type\":\"foundation.two_phase_fluid.two_phase_fluid\"}],\"Top\":[{\"id\":\"S\",\"label\":\"S\",\"type\":\"foundation.two_phase_fluid.two_phase_fluid\"}]}"
  Transfer Fcn : TransferFcn  Denominator=[1 1]
  Transfer Fcn1 : TransferFcn  Denominator=[0.5 1]
  Two-Phase Fluid R410a : SimscapeFluids_lib/Two-Phase Fluid/Utilities/Two-Phase Fluid Predefined Properties (2P)  fluid=fluids.two_phase_fluid.utilities.enum.Fluid.R410a  p_atm=0.101325 MPa  q_rev=0.01 Pa
  Water-Antifreeze Mix : SimscapeFluids_lib/Thermal Liquid/Utilities/Thermal Liquid Properties (TL)  fluid_list=fluids.thermal_liquid.utilities.enum.thermal_liquid_fluid_list.propylene_glycol  concentration_param_EG=fluids.thermal_liquid.utilities.enum.thermal_liquid_concentration.volume_fraction  concentration_param_PG=fluids.thermal_liquid.utilities.enum.thermal_liquid_concentration.mass_fraction  c_mass_SW=3.5e-3  c_mass_EG=0.1  c_mass_PG=0.12  c_mass_GL=0.1  c_vol_EG=0.1  c_vol_PG=0.1  beta_const_EG=2.1791 GPa  beta_const_PG=2.1791 GPa  beta_const_GL=2.1791 GPa  p_min_EG=0.01 MPa  p_min_PG=0.001 MPa  p_min_GL=0.01 MPa  p_max_EG=50 MPa  p_max_PG=50 MPa  p_max_GL=50 MPa  p_atm=0.101325 MPa
  ValveOutput : Outport  VectorParamsAs1DForOutWhenUnconnected=off
  S2_p : Outport  Port=2  VectorParamsAs1DForOutWhenUnconnected=off
  wires:
  [tAvg] -> Mux3/2
  Mux/1 -> Scope/1
  Mux2/1 -> Scope4/1
  PS-Simulink Converter6/1 -> Mux4/1  "p_G_B"
  Cycle Points/2(h) -> P-H Diagram (2P)/2
  PS-Simulink Converter5/1 -> Mux2/2  "t_G_A"
  Mux1/1 -> Scope2/1
  Mux4/1 -> Scope5/1
  PS-Simulink Converter1/1 -> Mux/2  "t_Eva_A"
  [tAtm] -> Mux3/1
  PS-Simulink Converter7/1 -> Mux2/1  "t_G_B"
  Temperature variation/1 -> House thermal network/1(tAtm), [tAtm]  "Ambient"
  Mux3/1 -> Scope1/1
  PS-Simulink Converter/1 -> Mux1/2  "p_Eva_A"
  PS-Simulink Converter2/1 -> Mux1/1  "p_Eva_B"
  PS-Simulink Converter8/1 -> Mux/1  "t_Eva_B"
  Cycle Points/1(p) -> P-H Diagram (2P)/1
  PS-Simulink Converter3/1 -> Scope3/1
  House thermal network/1(tAvg) -> [tAvg]  "Indoor average"
  PS-Simulink Converter4/1 -> Mux4/2  "p_G_A"
  [tAvg] -> ValveOutput/1
  [p2] -> S2_p/1
  Constant2/1 -> Switch/3
  [p2] -> Switch/2
  Constant1/1 -> Switch/1
  Transfer Fcn/1 -> Simulink-PS Converter/1
  ValveInput/1 -> Product/2
  Product/1 -> Transfer Fcn/1
  Switch/1 -> Transfer Fcn1/1
  Transfer Fcn1/1 -> Product/1
  connections:
  Heat Exchanger (TL-TL)/LConn2 -- Water-Antifreeze Mix/RConn1 -- Pressure & Temperature Sensor (TL)4/LConn1 -- Header Pipe 2/LConn1
  Condenser/RConn1 -- S2/LConn1 -- Compressor/RConn1
  Drive Ratio-CP/LConn1 -- Simulink-PS Converter/RConn1 -- Drive Ratio-DP/LConn1 -- Compressor/LConn2
  S1/RConn1 -- Compressor/LConn1 -- Accumulator/RConn1
  Pressure & Temperature Sensor (TL)1/LConn1 -- Evaporator/LConn1 -- Mass & Energy Flow Rate Sensor (TL)/RConn1
  Thermostatic Expansion Valve (2P)/RConn1 -- Evaporator/RConn1 -- S4/LConn1
  Flow Resistance (2P)/RConn1 -- Evaporator/RConn2 -- Thermostatic Expansion Valve (2P)/LConn2
  Header Pipe 1/RConn1 -- Local Restriction (TL)/LConn1 -- Pressure & Temperature Sensor (TL)2/LConn1
  Pressure & Temperature Sensor (TL)3/LConn1 -- Evaporator/LConn2 -- Ground loop pump/LConn1
  Solver Configuration/RConn1 -- S3/LConn1 -- Condenser/RConn2 -- Two-Phase Fluid R410a/RConn1 -- Thermostatic Expansion Valve (2P)/LConn1
  Distribution Pump/RConn1 -- House thermal network/LConn1
  Reservoir (TL)1/LConn1 -- Heat Exchanger (TL-TL)/RConn2
  Circulation Pump/LConn1 -- Hot Water Tank/LConn2
  Mass & Energy Flow Rate Sensor (TL)/RConn2 -- PS-Simulink Converter3/LConn1
  PS-Simulink Converter2/LConn1 -- Pressure & Temperature Sensor (TL)3/RConn2
  Mass Flow Rate Source (TL)/RConn1 -- Heat Exchanger (TL-TL)/RConn1
  Pressure & Temperature Sensor (TL)2/RConn2 -- PS-Simulink Converter4/LConn1
  Flow Resistance (2P)/LConn1 -- Accumulator/LConn1
  Heat Exchanger (TL-TL)/LConn1 -- Local Restriction (TL)/RConn1
  Pressure & Temperature Sensor (TL)3/RConn1 -- Absolute Reference (TL)3/LConn1
  PS-Simulink Converter8/LConn1 -- Pressure & Temperature Sensor (TL)3/RConn3
  Pressure & Temperature Sensor (TL)1/RConn2 -- PS-Simulink Converter/LConn1
  Pressure & Temperature Sensor (TL)2/RConn1 -- Absolute Reference (TL)2/LConn1
  Perfect Insulator3/LConn1 -- Header Pipe 2/LConn2
  PS-Simulink Converter5/LConn1 -- Pressure & Temperature Sensor (TL)2/RConn3
  Pressure & Temperature Sensor (TL)4/RConn1 -- Absolute Reference (TL)4/LConn1
  PS-Simulink Converter7/LConn1 -- Pressure & Temperature Sensor (TL)4/RConn3
  Drive Ratio-CP/RConn1 -- Circulation Pump/LConn2
  Perfect Insulator1/LConn1 -- Hot Water Tank/RConn2
  Hot Water Tank/LConn3 -- House thermal network/LConn2
  Condenser/LConn2 -- Hot Water Tank/LConn1
  Header Pipe 1/LConn1 -- Ground loop pump/RConn1
  Hot Water Tank/RConn1 -- Distribution Pump/LConn1
  Perfect Insulator/LConn1 -- Accumulator/LConn3
  Circulation Pump/RConn1 -- Condenser/LConn1
  Drive Ratio-DP/RConn1 -- Distribution Pump/LConn2
  Perfect Insulator4/LConn1 -- Header Pipe 1/LConn2
  PS-Simulink Converter1/LConn1 -- Pressure & Temperature Sensor (TL)1/RConn3
  Mass Flow Rate Source (TL)/LConn1 -- Reservoir (TL)/LConn1
  Cap (2P)1/LConn1 -- Accumulator/RConn2
  Pressure & Temperature Sensor (TL)1/RConn1 -- Absolute Reference (TL)1/LConn1
  Mass & Energy Flow Rate Sensor (TL)/LConn1 -- Header Pipe 2/RConn1
  Pump flow rate/RConn1 -- Ground loop pump/LConn2
  PS-Simulink Converter6/LConn1 -- Pressure & Temperature Sensor (TL)4/RConn2
  Cap (2P)/LConn1 -- Accumulator/LConn2

== system sm_DDPG_Training_Circuit_h4/Plant/Process ==
  note: Plant Model
      |
      | Capaci and Scali 2018 : Reproduction of Stiction model of valve
  Valve control : Inport
  Controlled_Flow : Outport  VectorParamsAs1DForOutWhenUnconnected=off
  wires:
  Valve control/1 -> Controlled_Flow/1

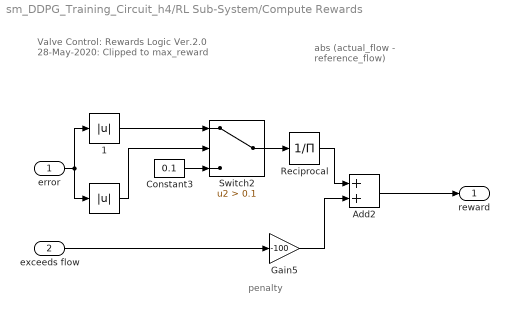
== system sm_DDPG_Training_Circuit_h4/RL Sub-System/Compute Rewards ==
  note: penalty
  note: abs (actual_flow - reference_flow)
  note: Valve Control: Rewards Logic
      | Ver.2.0 28-May-2020: Clipped to max_reward
  error : Inport
  exceeds flow : Inport  Port=2
  " " : Abs  SaturateOnIntegerOverflow=off
  " 1" : Abs  SaturateOnIntegerOverflow=off
  Add2 : Sum
  Constant3 : Constant  Value=0.1
  Gain5 : Gain  Gain=-100
  Reciprocal : Product  Inputs=/
  Switch2 : Switch  Criteria=u2 > Threshold  Threshold=0.1  SaturateOnIntegerOverflow=off  InputSameDT=off
  reward : Outport  VectorParamsAs1DForOutWhenUnconnected=off
  wires:
  Gain5/1 -> Add2/2
  exceeds flow/1 -> Gain5/1
  error/1 -> " 1"/1, " "/1
  " "/1 -> Switch2/2
  Reciprocal/1 -> Add2/1
  Switch2/1 -> Reciprocal/1
  Constant3/1 -> Switch2/3
  " 1"/1 -> Switch2/1
  Add2/1 -> reward/1

== system sm_DDPG_Training_Circuit_h4/RL Sub-System/Observation vector ==
  Actual flow : Inport
  Error signal : Inport  Port=2
  Discrete-Time Integrator : DiscreteIntegrator  SampleTime=Ts  ICPrevOutput=DiscIntNeverNeededParam  ICPrevScaledInput=DiscIntNeverNeededParam
  Mux1 : Mux  Inputs=3
  Observation vector : Outport  VectorParamsAs1DForOutWhenUnconnected=off
  wires:
  Discrete-Time Integrator/1 -> Mux1/3
  Mux1/1 -> Observation vector/1
  Error signal/1 -> Discrete-Time Integrator/1, Mux1/2
  Actual flow/1 -> Mux1/1

== system sm_DDPG_Training_Circuit_h4/RL Sub-System/Stop-simulation ==
  Actual flow : Inport
  s2_p : Inport  Port=2
  Compare To Constant : simulink/Logic and Bit Operations/Compare To Constant  relop=>  const=30  OutDataTypeStr=boolean
  Compare To Constant2 : simulink/Logic and Bit Operations/Compare To Constant  relop=<  const=5  OutDataTypeStr=boolean
  Compare To Constant3 : simulink/Logic and Bit Operations/Compare To Constant  relop=>=  const=5.65  OutDataTypeStr=boolean
  OR : Logic  Operator=OR  Inputs=3  IconShape=distinctive  AllPortsSameDT=off  OutDataTypeStr=boolean
  STOP : Outport  VectorParamsAs1DForOutWhenUnconnected=off
  wires:
  Compare To Constant/1 -> OR/1
  Actual flow/1 -> Compare To Constant/1, Compare To Constant2/1
  Compare To Constant2/1 -> OR/2
  OR/1 -> STOP/1
  s2_p/1 -> Compare To Constant3/1
  Compare To Constant3/1 -> OR/3

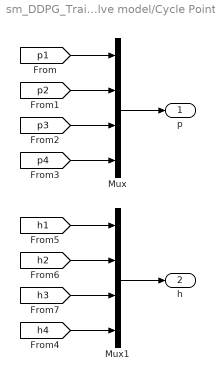
== system sm_DDPG_Training_Circuit_h4/Plant/Non-linear Valve model/Cycle Points ==
  Mux : Mux
  Mux1 : Mux
  p : Outport
  h : Outport  Port=2
  wires:
  [h1] -> Mux1/1
  [h2] -> Mux1/2
  [h3] -> Mux1/3
  [h4] -> Mux1/4
  [p1] -> Mux/1
  [p2] -> Mux/2
  [p3] -> Mux/3
  [p4] -> Mux/4
  Mux/1 -> p/1
  Mux1/1 -> h/1
